simulink subsystem "EKF_GyroIntegrator"  (R2021a)
settings: Solver=VariableStepAuto  StartTime=0.0  StopTime=10.0  RelTol=1e-3
undefined symbols (not defined in the file): Ts
libraries: dspmtrx3 x4, attitude_library x4
settings Model: Creator=Laura  LastModifiedBy=Laura

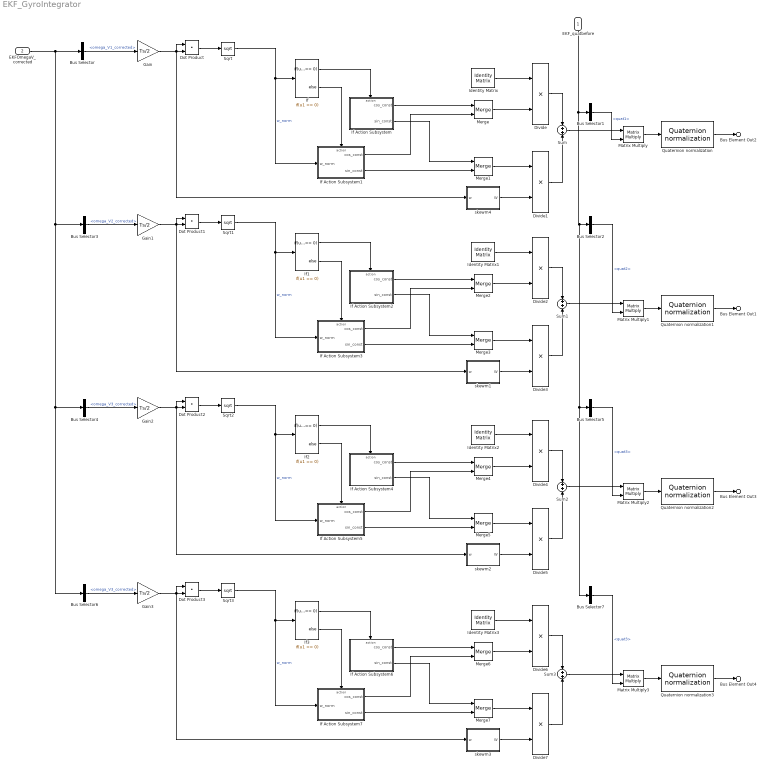
== system EKF_GyroIntegrator ==
  EKF_quatbefore : Inport
  EKFOmegaV_corrected : Inport  Port=2
  Bus Selector : BusSelector  OutputSignals=omega_V1_corrected
  Bus Selector1 : BusSelector  OutputSignals=quat1
  Bus Selector2 : BusSelector  OutputSignals=quat2
  Bus Selector3 : BusSelector  OutputSignals=omega_V2_corrected
  Bus Selector4 : BusSelector  OutputSignals=omega_V3_corrected
  Bus Selector5 : BusSelector  OutputSignals=quat3
  Bus Selector6 : BusSelector  OutputSignals=omega_V3_corrected
  Bus Selector7 : BusSelector  OutputSignals=quat3
  Divide{,1..7} (8 alike) : Product  Inputs=**
  Dot Product{,1..3} (4 alike) : DotProduct  InputSameDT=on  OutDataTypeStr=Inherit: Inherit via internal rule
  Gain{,1..3} (4 alike) : Gain  Gain=Ts/2
  Identity Matrix{,1..3} (4 alike) : dspmtrx3/Identity Matrix  Inherit=off  N=4  Ts=1  dataType=double  isSigned=on  wordLen=16  udDataType=sfix(16)  fracBitsMode=Best precision  numFracBits=15  OutDataTypeStr=double  LastOutDataTypeStr=double
  If{,1..3} (4 alike) : If  IfExpression=u1 == 0
  If Action Subsystem : Subsystem  TreatAsAtomicUnit=on
  If Action Subsystem1 : Subsystem  TreatAsAtomicUnit=on
  If Action Subsystem2 : Subsystem  TreatAsAtomicUnit=on
  If Action Subsystem3 : Subsystem  TreatAsAtomicUnit=on
  If Action Subsystem4 : Subsystem  TreatAsAtomicUnit=on
  If Action Subsystem5 : Subsystem  TreatAsAtomicUnit=on
  If Action Subsystem6 : Subsystem  TreatAsAtomicUnit=on
  If Action Subsystem7 : Subsystem  TreatAsAtomicUnit=on
  Matrix Multiply{,1..3} (4 alike) : Product  Multiplication=Matrix(*)
  Merge{,1..7} (8 alike) : Merge
  Quaternion normalization{,1..3} (4 alike) : attitude_library/Quaternion normalization  SystemSampleTime=-1  VariantActivationTime=update diagram  Latency=0  AutoFrameSizeCalculation=off
      settings: SourceProductName=Attitude library
  Sqrt{,1..3} (4 alike) : Sqrt  SaturateOnIntegerOverflow=on
  Sum{,1..3} (4 alike) : Sum
  skewm1 : MATLAB Function  TreatAsAtomicUnit=on
  skewm2 : MATLAB Function  TreatAsAtomicUnit=on
  skewm3 : MATLAB Function  TreatAsAtomicUnit=on
  skewm4 : MATLAB Function  TreatAsAtomicUnit=on
  Bus Element Out2 : Outport  PortName=EKF_quatprop  Element=quat1
  Bus Element Out1 : Outport  PortName=EKF_quatprop  Element=quat2
  Bus Element Out3 : Outport  PortName=EKF_quatprop  Element=quat3
  Bus Element Out4 : Outport  PortName=EKF_quatprop  Element=quat4
  wires:
  Divide7/1 -> Sum3/2
  Divide6/1 -> Sum3/1
  Sum3/1 -> Matrix Multiply3/1
  EKF_quatbefore/1 -> Bus Selector7/1, Bus Selector5/1, Bus Selector2/1, Bus Selector1/1
  Quaternion normalization3/1 -> Bus Element Out4/1
  Matrix Multiply3/1 -> Quaternion normalization3/1
  Bus Selector7/1 -> Matrix Multiply3/2  "<quat3>"
  Merge7/1 -> Divide7/1
  Sqrt3/1 -> If Action Subsystem7/1(w_norm), If3/1  "w_norm"
  Merge6/1 -> Divide6/2
  Bus Selector6/1 -> Gain3/1  "<omega_V3_corrected>"
  Gain3/1 -> skewm3/1(w), Dot Product3/2, Dot Product3/1
  skewm3/1(W) -> Divide7/2
  Identity Matrix3/1 -> Divide6/1
  If3/2 -> If Action Subsystem7/Action
  If Action Subsystem7/2(sin_const) -> Merge7/2
  If Action Subsystem7/1(cos_const) -> Merge6/2
  If Action Subsystem6/2(sin_const) -> Merge7/1
  Dot Product3/1 -> Sqrt3/1
  If3/1 -> If Action Subsystem6/Action
  If Action Subsystem6/1(cos_const) -> Merge6/1
  Gain2/1 -> skewm2/1(w), Dot Product2/2, Dot Product2/1
  Sqrt2/1 -> If Action Subsystem5/1(w_norm), If2/1  "w_norm"
  If Action Subsystem5/2(sin_const) -> Merge5/2
  If Action Subsystem4/1(cos_const) -> Merge4/1
  If Action Subsystem5/1(cos_const) -> Merge4/2
  If2/2 -> If Action Subsystem5/Action
  Merge5/1 -> Divide5/1
  If Action Subsystem4/2(sin_const) -> Merge5/1
  Divide4/1 -> Sum2/1
  skewm2/1(W) -> Divide5/2
  Divide5/1 -> Sum2/2
  Identity Matrix2/1 -> Divide4/1
  Bus Selector4/1 -> Gain2/1  "<omega_V3_corrected>"
  If2/1 -> If Action Subsystem4/Action
  Merge4/1 -> Divide4/2
  Dot Product2/1 -> Sqrt2/1
  Matrix Multiply2/1 -> Quaternion normalization2/1
  Bus Selector5/1 -> Matrix Multiply2/2  "<quat3>"
  Quaternion normalization2/1 -> Bus Element Out3/1
  Sum2/1 -> Matrix Multiply2/1
  Bus Selector3/1 -> Gain1/1  "<omega_V2_corrected>"
  EKFOmegaV_corrected/1 -> Bus Selector6/1, Bus Selector4/1, Bus Selector3/1, Bus Selector/1
  skewm1/1(W) -> Divide3/2
  Dot Product1/1 -> Sqrt1/1
  Sqrt1/1 -> If Action Subsystem3/1(w_norm), If1/1  "w_norm"
  Identity Matrix1/1 -> Divide2/1
  If Action Subsystem2/2(sin_const) -> Merge3/1
  Divide2/1 -> Sum1/1
  Merge3/1 -> Divide3/1
  If Action Subsystem3/2(sin_const) -> Merge3/2
  If Action Subsystem2/1(cos_const) -> Merge2/1
  If Action Subsystem3/1(cos_const) -> Merge2/2
  If1/2 -> If Action Subsystem3/Action
  Divide3/1 -> Sum1/2
  Gain1/1 -> skewm1/1(w), Dot Product1/2, Dot Product1/1
  If1/1 -> If Action Subsystem2/Action
  Merge2/1 -> Divide2/2
  Bus Selector2/1 -> Matrix Multiply1/2  "<quat2>"
  Matrix Multiply1/1 -> Quaternion normalization1/1
  Quaternion normalization1/1 -> Bus Element Out1/1
  Sum1/1 -> Matrix Multiply1/1
  Bus Selector/1 -> Gain/1  "<omega_V1_corrected>"
  Bus Selector1/1 -> Matrix Multiply/2  "<quat1>"
  Quaternion normalization/1 -> Bus Element Out2/1
  Gain/1 -> skewm4/1(w), Dot Product/2, Dot Product/1
  Dot Product/1 -> Sqrt/1
  Sqrt/1 -> If Action Subsystem1/1(w_norm), If/1  "w_norm"
  If/1 -> If Action Subsystem/Action
  If/2 -> If Action Subsystem1/Action
  If Action Subsystem/1(cos_const) -> Merge/1
  If Action Subsystem1/1(cos_const) -> Merge/2
  If Action Subsystem/2(sin_const) -> Merge1/1
  If Action Subsystem1/2(sin_const) -> Merge1/2
  Merge/1 -> Divide/2
  Identity Matrix/1 -> Divide/1
  skewm4/1(W) -> Divide1/2
  Merge1/1 -> Divide1/1
  Divide/1 -> Sum/1
  Divide1/1 -> Sum/2
  Sum/1 -> Matrix Multiply/1
  Matrix Multiply/1 -> Quaternion normalization/1

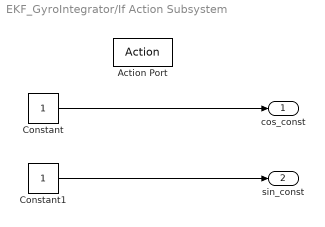
== system EKF_GyroIntegrator/If Action Subsystem ==
  Action Port : ActionPort
  Constant : Constant
  Constant1 : Constant
  cos_const : Outport
  sin_const : Outport  Port=2
  wires:
  Constant1/1 -> sin_const/1
  Constant/1 -> cos_const/1

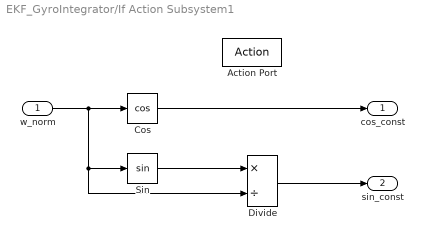
== system EKF_GyroIntegrator/If Action Subsystem1 ==
  w_norm : Inport
  Action Port : ActionPort
  Cos : Trigonometry  Operator=cos
  Divide : Product  Inputs=*/
  Sin : Trigonometry
  cos_const : Outport
  sin_const : Outport  Port=2
  wires:
  Cos/1 -> cos_const/1
  Divide/1 -> sin_const/1
  w_norm/1 -> Divide/2, Sin/1, Cos/1
  Sin/1 -> Divide/1

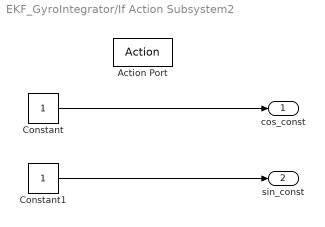
== system EKF_GyroIntegrator/If Action Subsystem2 ==
  Action Port : ActionPort
  Constant : Constant
  Constant1 : Constant
  cos_const : Outport
  sin_const : Outport  Port=2
  wires:
  Constant1/1 -> sin_const/1
  Constant/1 -> cos_const/1

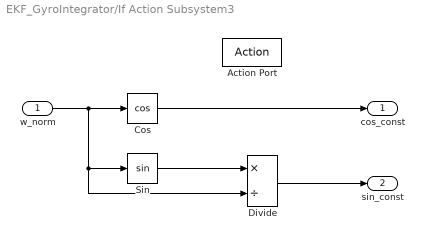
== system EKF_GyroIntegrator/If Action Subsystem3 ==
  w_norm : Inport
  Action Port : ActionPort
  Cos : Trigonometry  Operator=cos
  Divide : Product  Inputs=*/
  Sin : Trigonometry
  cos_const : Outport
  sin_const : Outport  Port=2
  wires:
  Cos/1 -> cos_const/1
  Divide/1 -> sin_const/1
  w_norm/1 -> Divide/2, Sin/1, Cos/1
  Sin/1 -> Divide/1

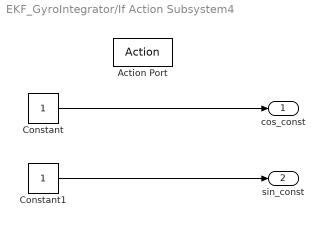
== system EKF_GyroIntegrator/If Action Subsystem4 ==
  Action Port : ActionPort
  Constant : Constant
  Constant1 : Constant
  cos_const : Outport
  sin_const : Outport  Port=2
  wires:
  Constant1/1 -> sin_const/1
  Constant/1 -> cos_const/1

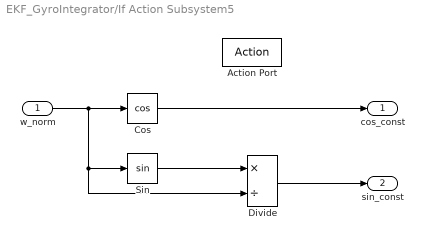
== system EKF_GyroIntegrator/If Action Subsystem5 ==
  w_norm : Inport
  Action Port : ActionPort
  Cos : Trigonometry  Operator=cos
  Divide : Product  Inputs=*/
  Sin : Trigonometry
  cos_const : Outport
  sin_const : Outport  Port=2
  wires:
  Cos/1 -> cos_const/1
  Divide/1 -> sin_const/1
  w_norm/1 -> Divide/2, Sin/1, Cos/1
  Sin/1 -> Divide/1

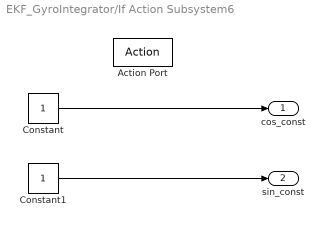
== system EKF_GyroIntegrator/If Action Subsystem6 ==
  Action Port : ActionPort
  Constant : Constant
  Constant1 : Constant
  cos_const : Outport
  sin_const : Outport  Port=2
  wires:
  Constant1/1 -> sin_const/1
  Constant/1 -> cos_const/1

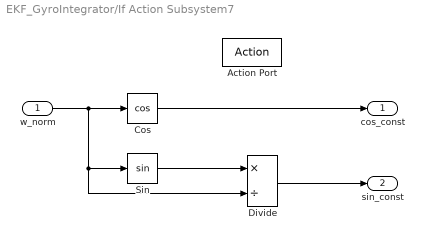
== system EKF_GyroIntegrator/If Action Subsystem7 ==
  w_norm : Inport
  Action Port : ActionPort
  Cos : Trigonometry  Operator=cos
  Divide : Product  Inputs=*/
  Sin : Trigonometry
  cos_const : Outport
  sin_const : Outport  Port=2
  wires:
  Cos/1 -> cos_const/1
  Divide/1 -> sin_const/1
  w_norm/1 -> Divide/2, Sin/1, Cos/1
  Sin/1 -> Divide/1

== matlab function EKF_GyroIntegrator/skewm1 ==
  data: w input; W output
function W = skewm4(w)
% skewm forms a skew-symmetric 4x4 matrix from a 3x1 vector
%
% INPUT
%              w, 3x1 vector
%
%	OUTPUT
%              W, 4x4 skew-symmetric matrix
%
%%
%     W=[  0  w(3)  -w(2)  w(1);
%        -w(3)    0  w(1)  w(2);
%         w(2) -w(1)   0   w(3);
%        -w(1) -w(2) -w(3)    0];
   
       W=[  0  -w(1)  -w(2)  -w(3);
          w(1)    0    w(3)  -w(2);
          w(2) -w(3)     0    w(1);
          w(3)  w(2)  -w(1)     0];
   
end

== matlab function EKF_GyroIntegrator/skewm2 ==
  data: w input; W output
function W = skewm4(w)
% skewm forms a skew-symmetric 4x4 matrix from a 3x1 vector
%
% INPUT
%              w, 3x1 vector
%
%	OUTPUT
%              W, 4x4 skew-symmetric matrix
%
%%
%     W=[  0  w(3)  -w(2)  w(1);
%        -w(3)    0  w(1)  w(2);
%         w(2) -w(1)   0   w(3);
%        -w(1) -w(2) -w(3)    0];
   
       W=[  0  -w(1)  -w(2)  -w(3);
          w(1)    0    w(3)  -w(2);
          w(2) -w(3)     0    w(1);
          w(3)  w(2)  -w(1)     0];
   
end

== matlab function EKF_GyroIntegrator/skewm3 ==
  data: w input; W output
function W = skewm4(w)
% skewm forms a skew-symmetric 4x4 matrix from a 3x1 vector
%
% INPUT
%              w, 3x1 vector
%
%	OUTPUT
%              W, 4x4 skew-symmetric matrix
%
%%
%     W=[  0  w(3)  -w(2)  w(1);
%        -w(3)    0  w(1)  w(2);
%         w(2) -w(1)   0   w(3);
%        -w(1) -w(2) -w(3)    0];
   
       W=[  0  -w(1)  -w(2)  -w(3);
          w(1)    0    w(3)  -w(2);
          w(2) -w(3)     0    w(1);
          w(3)  w(2)  -w(1)     0];
   
end

== matlab function EKF_GyroIntegrator/skewm4 ==
  data: w input; W output
function W = skewm4(w)
% skewm forms a skew-symmetric 4x4 matrix from a 3x1 vector
%
% INPUT
%              w, 3x1 vector
%
%	OUTPUT
%              W, 4x4 skew-symmetric matrix
%
%%
%     W=[  0  w(3)  -w(2)  w(1);
%        -w(3)    0  w(1)  w(2);
%         w(2) -w(1)   0   w(3);
%        -w(1) -w(2) -w(3)    0];
   
       W=[  0  -w(1)  -w(2)  -w(3);
          w(1)    0    w(3)  -w(2);
          w(2) -w(3)     0    w(1);
          w(3)  w(2)  -w(1)     0];
   
end
